simulink model "Aerobic_tank_model"  (R2023a)
settings: Solver=VariableStepAuto  StartTime=0.0  StopTime=10.0  RelTol=1e-3
model workspace (MAT data in the model file):
  Q0 = Simulink.Parameter
  Q0.DataType = 'auto'
  Q0.Complexity = 'real'
  Q0.Dimensions = [0 0]
values from neighbouring files (symbols this model uses):
  iXB = 0.08    [Start2.m]
  iXP = 0.06    [Start2.m]
  kLa = 240    [Start2.m]
  Q1 = 55000    [Start2.m]
  Qa = 10000    [Start2.m]
  Qr = 20000    [Start2.m]
  SALK0 = InputSediments(13)    [Start2.m]
  SALK_ini = 4.93    [Start2.m]
  SALK_ini2 = 4.67    [Start2.m]
  SI0 = InputSediments(1)    [Start2.m]
  SI_ini = 30    [Start2.m]
  SI_ini2 = 30    [Start2.m]
  SND0 = InputSediments(11)    [Start2.m]
  SND_ini = 1.22    [Start2.m]
  SND_ini2 = 0.82    [Start2.m]
  SNH0 = InputSediments(10)    [Start2.m]
  SNH_ini = 7.92    [Start2.m]
  SNH_ini2 = 5.55    [Start2.m]
  SNO0 = InputSediments(9)    [Start2.m]
  SNO_ini = 5.37    [Start2.m]
  SNO_ini2 = 6.54    [Start2.m]
  SO0 = InputSediments(8)    [Start2.m]
  SO_ini = 0.004    [Start2.m]
  SO_ini2 = 1.7    [Start2.m]
  SRT = 100    [Start2.m]
  SS0 = InputSediments(2)    [Start2.m]
  SS_ini = 2.81    [Start2.m]
  SS_ini2 = 1.15    [Start2.m]
  V1 = 1000    [Start2.m]
  XBA0 = InputSediments(6)    [Start2.m]
  XBA_ini = 148    [Start2.m]
  XBA_ini2 = 150    [Start2.m]
  XBH0 = InputSediments(5)    [Start2.m]
  XBH_ini = 2552    [Start2.m]
  XBH_ini2 = 2559    [Start2.m]
  XI0 = InputSediments(3)    [Start2.m]
  XI_ini = 1149    [Start2.m]
  XI_ini2 = 1149    [Start2.m]
  XND0 = InputSediments(12)    [Start2.m]
  XND_ini = 5.28    [Start2.m]
  XND_ini2 = 4.39    [Start2.m]
  XP0 = InputSediments(7)    [Start2.m]
  XP_ini = 449    [Start2.m]
  XP_ini2 = 450    [Start2.m]
  XS0 = InputSediments(4)    [Start2.m]
  XS_ini = 82.1    [Start2.m]
  XS_ini2 = 64.9    [Start2.m]
settings Model: Creator=carlo  LastModifiedBy=carlo

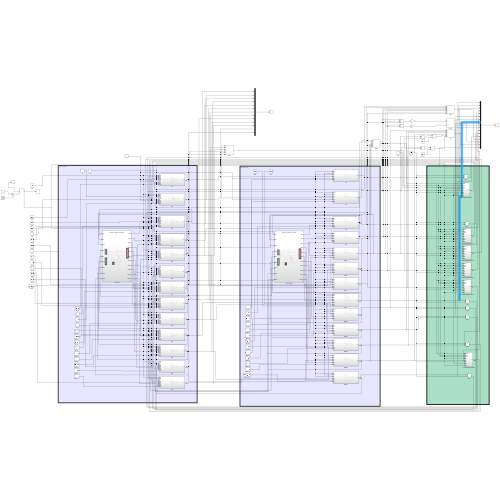
[thumbnail: Simulink's stored preview of the top-level diagram]
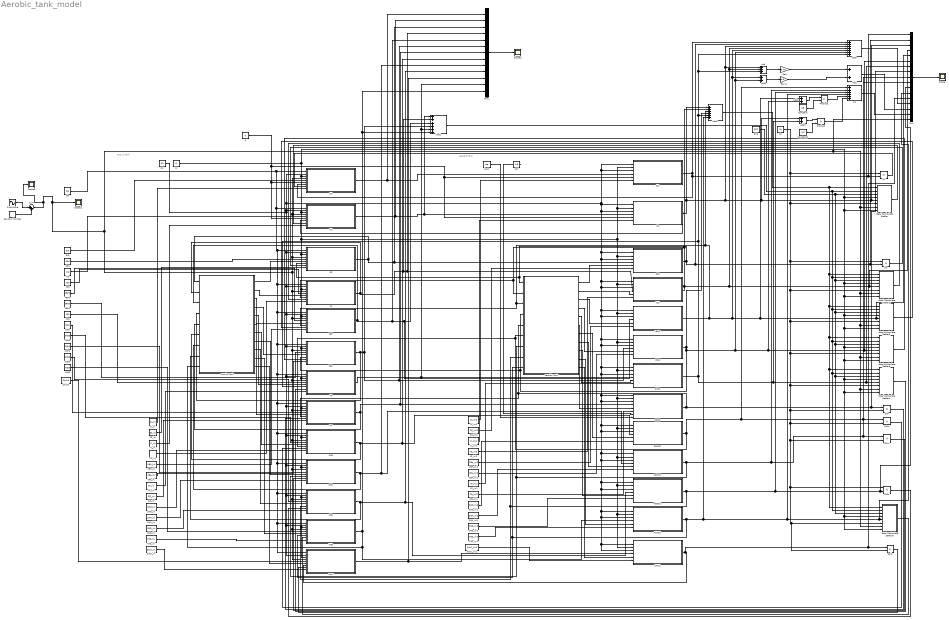
== system Aerobic_tank_model ==
  note: Aerated Tank
  note: Anoxic Tank
  0 : Constant  Value=0
  Add : Sum  Inputs=+++
  Add1 : Sum
  Add2 : Sum
  Add3 : Sum
  Aerobic Tank : Subsystem  ReferencedSubsystem=dynamic_models_processes
  Anoxic Tank : Subsystem  ReferencedSubsystem=dynamic_models_processes
  COD : Sum  Inputs=7
  Constant : Constant  Value=iXB
  Constant1 : Constant  Value=iXP
  Gain : Gain  Gain=0.75
  Gain1 : Gain  Gain=0.9
  Ideal Particulate Settler : Subsystem
  Ideal Particulate Settler1 : Subsystem
  Ideal Particulate Settler2 : Subsystem
  Ideal Particulate Settler3 : Subsystem
  Ideal Particulate Settler4 : Subsystem
  Ideal Particulate Settler5 : Subsystem
  Mux : Mux  Inputs=17
  Mux1 : Mux  Inputs=13
  Product : Product
  Product1 : Product
  Q1 : Constant  Value=Q1
  Qa : Constant  Value=Qa
  Qr : Constant  Value=Qr
  RSND2 : Subsystem
  RSNH2 : Subsystem
  RSNO2 : Subsystem
  RSO2 : Subsystem
  RXND2 : Subsystem
  RXP2 : Subsystem
  Random Number : RandomNumber  Mean=2000  Variance=250000  SampleTime=0.1
  SALK : Subsystem
  SALK0 : Constant  Value=SALK0
  SALK2 : Subsystem
  SALK_ini : Constant  Value=SALK_ini
  SALK_ini1 : Constant  Value=SALK_ini2
  SI0 : Constant  Value=SI0
  SI1 : Subsystem
  SI2 : Subsystem
  SI_ini : Constant  Value=SI_ini
  SI_ini2 : Constant  Value=SI_ini2
  SIr : Product
  SND : Subsystem
  SND0 : Constant  Value=SND0
  SND_ini : Constant  Value=SND_ini
  SND_ini1 : Constant  Value=SND_ini2
  SNDr : Product
  SNH : Subsystem
  SNH0 : Constant  Value=SNH0
  SNH_ini : Constant  Value=SNH_ini
  SNH_ini1 : Constant  Value=SNH_ini2
  SNHr : Product
  SNO : Subsystem
  SNO0 : Constant  Value=SNO0
  SNO_ini : Constant  Value=SNO_ini
  SNO_ini1 : Constant  Value=SNO_ini2
  SNOr : Product
  SO : Subsystem
  SO* : Constant  Value=0.8
  SO0 : Constant  Value=SO0
  SO_ini : Constant  Value=SO_ini
  SO_ini1 : Constant  Value=SO_ini2
  SOr : Product
  SS : Subsystem
  SS0 : Constant  Value=SS0
  SS2 : Subsystem
  SS_ini : Constant  Value=SS_ini
  SS_ini1 : Constant  Value=SS_ini2
  STR : Constant  Value=SRT
  Salkr : Product
  Scope{,1..3} (4 alike) : Scope
  Sine Wave : Sin  Amplitude=10000  Bias=20000  Frequency=2*pi  SampleTime=0
  Ssr : Product
  Sum : Sum  Inputs=|++
  TN : Sum  Inputs=6
  TSS : Sum  Inputs=2
  V1 : Constant  Value=V1
  XBA : Subsystem
  XBA0 : Constant  Value=XBA0
  XBA2 : Subsystem
  XBA_ini : Constant  Value=XBA_ini
  XBA_ini1 : Constant  Value=XBA_ini2
  XBH : Subsystem
  XBH0 : Constant  Value=XBH0
  XBH2 : Subsystem
  XBH_ini : Constant  Value=XBH_ini
  XBH_ini1 : Constant  Value=XBH_ini2
  XI0 : Constant  Value=XI0
  XI1 : Subsystem
  XI2 : Subsystem
  XI_ini : Constant  Value=XI_ini
  XI_ini2 : Constant  Value=XI_ini2
  XND : Subsystem
  XND0 : Constant  Value=XND0
  XND_ini : Constant  Value=XND_ini
  XND_ini1 : Constant  Value=XND_ini2
  XP : Subsystem
  XP0 : Constant  Value=XP0
  XP_ini : Constant  Value=XP_ini
  XP_ini1 : Constant  Value=XP_ini2
  XS : Subsystem
  XS0 : Constant  Value=XS0
  XS2 : Subsystem
  XS_ini : Constant  Value=XS_ini
  XS_ini1 : Constant  Value=XS_ini2
  Xtot1 : Sum  Inputs=6
  Xtot2 : Sum  Inputs=6
  kLa2 : Constant  Value=kLa
  wires:
  V1/1 -> Ideal Particulate Settler1/4(V1), Ideal Particulate Settler3/4(V1), Ideal Particulate Settler3/8(V2), Ideal Particulate Settler5/8(V2), Ideal Particulate Settler5/4(V1), Ideal Particulate Settler4/8(V2), Ideal Particulate Settler4/4(V1), Ideal Particulate Settler2/8(V2), Ideal Particulate Settler2/4(V1), Ideal Particulate Settler1/8(V2), Ideal Particulate Settler/8(V2), Ideal Particulate Settler/4(V1), SNH/3(V1), SALK/3(V1), XND/3(V1), SND/3(V1), SNO/3(V1), SO/3(V1), XP/3(V1), XBA/3(V1), XBH/3(V1), XS/3(V1), SS/3(V1), XI2/2(V2), SI2/2(V2), SALK2/2(V2), RXND2/2(V2), RSND2/2(V2), RSNH2/2(V2), RSNO2/2(V2), RSO2/2(V2), RXP2/2(V2), XBA2/2(V2), XBH2/2(V2), XS2/2(V2), SS2/2(V2), XI1/3(V1), SI1/3(V1)
  Q1/1 -> SALK/2(Q1), XND/2(Q1), SND/2(Q1), SNH/2(Q1), SNO/2(Q1), SO/2(Q1), XP/2(Q1), XBA/2(Q1), XBH/2(Q1), XS/2(Q1), SS/2(Q1), SI1/2(Q1), SS2/3(Q1), SALK2/3(Q1), SALK2/1(Q2), RXND2/3(Q1), RXND2/1(Q2), RSND2/3(Q1), RSND2/1(Q2), RSNH2/3(Q1), RSNH2/1(Q2), RSNO2/3(Q1), RSNO2/1(Q2), RSO2/3(Q1), RSO2/1(Q2), RXP2/3(Q1), RXP2/1(Q2), XBA2/3(Q1), XBA2/1(Q2), XBH2/3(Q1), XBH2/1(Q2), XS2/3(Q1), XS2/1(Q2), SS2/1(Q2), XI2/3(Q1), XI2/1(Q2), SI2/1(Q2), SI2/3(Q1), XI1/2(Q1)
  Sum/1 -> Scope3/1, XBH/4(Q0), SO/4(Q0), SNH/4(Q0), XND/4(Q0), SALK/4(Q0), SND/4(Q0), SNO/4(Q0), XP/4(Q0), XBA/4(Q0), XS/4(Q0), XI1/4(Q0), SI1/4(Q0), SS/4(Q0), Mux/17, Ideal Particulate Settler/7(Q0), Ideal Particulate Settler5/7(Q0), Ideal Particulate Settler4/7(Q0), Ideal Particulate Settler3/7(Q0), Ideal Particulate Settler2/7(Q0), Ideal Particulate Settler1/7(Q0), Scope1/1
  Anoxic Tank/1 -> SS/6(R1)
  SS/1(Z1) -> Mux1/3, SS2/4(Z1), Anoxic Tank/1  "SS1"
  XP0/1 -> XP/5(Z0)
  SNO0/1 -> SNO/5(Z0)
  SND0/1 -> SND/5(Z0)
  SALK0/1 -> SALK/5(Z0)
  Anoxic Tank/2 -> XS/6(R1)
  Anoxic Tank/3 -> XBH/6(R1)
  Anoxic Tank/4 -> XBA/6(R1)
  Anoxic Tank/5 -> XP/6(R1)
  Anoxic Tank/6 -> SO/6(R1)
  Anoxic Tank/7 -> SNO/6(R1)
  Anoxic Tank/8 -> SNH/6(R1)
  Anoxic Tank/9 -> SND/6(R1)
  Anoxic Tank/10 -> XND/6(R1)
  Anoxic Tank/11 -> SALK/6(R1)
  XS/1(Z1) -> Xtot1/2, Mux1/4, XS2/4(Z1), Anoxic Tank/2  "XS1"
  XBH/1(Z1) -> Mux1/5, Xtot1/3, XBH2/4(Z1), Anoxic Tank/3  "XBH1"
  XBA/1(Z1) -> Xtot1/4, Mux1/6, XBA2/4(Z1), Anoxic Tank/4  "XBA1"
  XP/1(Z1) -> RXP2/4(Z1), Mux1/12, Xtot1/5  "XP1"
  SO/1(Z1) -> Anoxic Tank/5, Mux1/7, RSO2/4(Z1)  "SO1"
  SNO/1(Z1) -> Anoxic Tank/6, Mux1/8, RSNO2/4(Z1)  "SNO1"
  SNH/1(Z1) -> Anoxic Tank/7, Mux1/9, RSNH2/4(Z1)  "SNH1"
  SND/1(Z1) -> Anoxic Tank/8, Mux1/10, RSND2/4(Z1)  "SND1"
  XND/1(Z1) -> Mux1/13, Xtot1/6, RXND2/4(Z1), Anoxic Tank/9  "XND1"
  SALK/1(Z1) -> Mux1/11, SALK2/4(Z1)  "SALK1"
  SS_ini/1 -> SS/9(Zini)
  XS_ini/1 -> XS/9(Zini)
  XBH_ini/1 -> XBH/9(Zini)
  XBA_ini/1 -> XBA/9(Zini)
  XP_ini/1 -> XP/9(Zini)
  SO_ini/1 -> SO/9(Zini)
  SNO_ini/1 -> SNO/9(Zini)
  SNH_ini/1 -> SNH/9(Zini)
  SND_ini/1 -> SND/9(Zini)
  XND_ini/1 -> XND/9(Zini)
  SALK_ini/1 -> SALK/9(Zini)
  SS2/1(Z2) -> Mux/2, Ssr/2, COD/2, SS/7(Za), Aerobic Tank/1  "SS2"
  XS2/1(Z2) -> Mux/4, Ideal Particulate Settler1/5(X), Add/2, COD/4, Xtot2/2, XS/7(Za), Aerobic Tank/2
  XBH2/1(Z2) -> Add2/1, Mux/5, Ideal Particulate Settler2/5(X), Add1/1, COD/5, Xtot2/3, XBH/7(Za), Aerobic Tank/3
  XBA2/1(Z2) -> Xtot2/4, XBA/7(Za), Aerobic Tank/4, Add2/2, Ideal Particulate Settler3/5(X), Mux/6, COD/6, Add1/2  "XBA2"
  kLa2/1 -> RSO2/8(kLa)
  SO*/1 -> RSO2/7(SO*)
  RSO2/1(Z2) -> SOr/1, Mux/8, Aerobic Tank/5, SO/7(Za)  "SO2"
  RSNO2/1(Z2) -> TN/1, SNOr/1, Mux/9, Aerobic Tank/6, SNO/7(Za)  "SNO2"
  RSNH2/1(Z2) -> TN/2, SNHr/1, Mux/10, SNH/7(Za), Aerobic Tank/7  "SNH2"
  RSND2/1(Z2) -> TN/3, Mux/11, SNDr/2, SND/7(Za), Aerobic Tank/8  "SND2"
  RXND2/1(Z2) -> Xtot2/6, TN/4, Mux/12, Ideal Particulate Settler5/5(X), XND/7(Za), Aerobic Tank/9  "XND2"
  Aerobic Tank/2 -> XS2/5(R2)
  Aerobic Tank/3 -> XBH2/5(R2)
  Aerobic Tank/4 -> XBA2/5(R2)
  Aerobic Tank/5 -> RXP2/5(R2)
  Aerobic Tank/6 -> RSO2/5(R2)
  Aerobic Tank/7 -> RSNO2/5(R2)
  Aerobic Tank/8 -> RSNH2/5(R2)
  Aerobic Tank/9 -> RSND2/5(R2)
  Aerobic Tank/10 -> RXND2/5(R2)
  Aerobic Tank/11 -> SALK2/5(R2)
  Aerobic Tank/1 -> SS2/5(R2)
  SS_ini1/1 -> SS2/6(Zini)
  XS_ini1/1 -> XS2/6(Zini)
  XBH_ini1/1 -> XBH2/6(Zini)
  XBA_ini1/1 -> XBA2/6(Zini)
  XP_ini1/1 -> RXP2/6(Zini)
  SO_ini1/1 -> RSO2/6(Zini)
  SNO_ini1/1 -> RSNO2/6(Zini)
  SNH_ini1/1 -> RSNH2/6(Zini)
  SND_ini1/1 -> RSND2/6(Zini)
  XND_ini1/1 -> RXND2/6(Zini)
  SALK_ini1/1 -> SALK2/6(Zini)
  SALK2/1(Z2) -> Salkr/1, Mux/13, SALK/7(Za)  "SALK2"
  RXP2/1(Z2) -> Add/3, COD/7, Xtot2/5, XP/7(Za), Add3/2, Ideal Particulate Settler4/5(X), Mux/7  "XP2"
  0/1 -> XI1/6(R1), SI1/6(R1), SI2/5(R2), XI2/5(R2)
  SI0/1 -> SI1/5(Z0)
  SI_ini/1 -> SI1/9(Zini)
  XI_ini/1 -> XI1/9(Zini)
  SI1/1(Z1) -> Mux1/1, SI2/4(Z1)  "SI1"
  XI1/1(Z1) -> Mux1/2, Xtot1/1, XI2/4(Z1)  "XI1"
  SI_ini2/1 -> SI2/6(Zini)
  XI_ini2/1 -> XI2/6(Zini)
  SI2/1(Z2) -> COD/1, SIr/2, Mux/1, SI1/7(Za)
  XI2/1(Z2) -> XI1/7(Za), COD/3, Add/1, Add3/1, Mux/3, Ideal Particulate Settler/5(X), Xtot2/1
  Qr/1 -> Salkr/2, Ideal Particulate Settler5/6(Qr), SNDr/1, SNHr/2, SNOr/2, SOr/2, Ideal Particulate Settler4/6(Qr), Ideal Particulate Settler3/6(Qr), Ideal Particulate Settler2/6(Qr), Ideal Particulate Settler1/6(Qr), Ssr/1, Ideal Particulate Settler/6(Qr), SIr/1
  Xtot2/1 -> Ideal Particulate Settler/1(Xtot2), Ideal Particulate Settler5/1(Xtot2), Ideal Particulate Settler4/1(Xtot2), Ideal Particulate Settler3/1(Xtot2), Ideal Particulate Settler2/1(Xtot2), Ideal Particulate Settler1/1(Xtot2)
  Xtot1/1 -> Ideal Particulate Settler/2(Xtot1), Ideal Particulate Settler5/2(Xtot1), Ideal Particulate Settler4/2(Xtot1), Ideal Particulate Settler3/2(Xtot1), Ideal Particulate Settler2/2(Xtot1), Ideal Particulate Settler1/2(Xtot1)
  STR/1 -> Ideal Particulate Settler/3(STR), Ideal Particulate Settler5/3(STR), Ideal Particulate Settler4/3(STR), Ideal Particulate Settler3/3(STR), Ideal Particulate Settler2/3(STR), Ideal Particulate Settler1/3(STR)
  Ideal Particulate Settler1/1(Zr) -> XS/8(Zr)  "XSr"
  Ideal Particulate Settler2/1(Zr) -> XBH/8(Zr)  "XBHr"
  Ideal Particulate Settler3/1(Zr) -> XBA/8(Zr)  "XBAr"
  Ideal Particulate Settler5/1(Zr) -> XND/8(Zr)  "XNDr"
  SIr/1 -> SI1/8(Zr)
  Ideal Particulate Settler/1(Zr) -> XI1/8(Zr)  "XIr"
  Ssr/1 -> SS/8(Zr)
  Ideal Particulate Settler4/1(Zr) -> XP/8(Zr)  "XPr"
  SOr/1 -> SO/8(Zr)
  SNOr/1 -> SNO/8(Zr)
  SNHr/1 -> SNH/8(Zr)
  SNDr/1 -> SND/8(Zr)
  Salkr/1 -> SALK/8(Zr)
  Qa/1 -> SNH/1(Qa), SALK/1(Qa), XND/1(Qa), SND/1(Qa), SNO/1(Qa), SO/1(Qa), XP/1(Qa), XBA/1(Qa), XBH/1(Qa), XS/1(Qa), SS/1(Qa), XI1/1(Qa), SI1/1(Qa)
  SS0/1 -> SS/5(Z0)
  XI0/1 -> XI1/5(Z0)
  XS0/1 -> XS/5(Z0)
  XBH0/1 -> XBH/5(Z0)
  XBA0/1 -> XBA/5(Z0)
  SO0/1 -> SO/5(Z0)
  SNH0/1 -> SNH/5(Z0)
  XND0/1 -> XND/5(Z0)
  Add/1 -> Gain/1
  Add1/1 -> Gain1/1
  Gain/1 -> TSS/1
  Gain1/1 -> TSS/2
  Constant/1 -> Product1/2
  Add2/1 -> Product1/1
  Product1/1 -> TN/5
  Add3/1 -> Product/1
  Constant1/1 -> Product/2
  Product/1 -> TN/6
  COD/1 -> Mux/14
  TSS/1 -> Mux/15
  TN/1 -> Mux/16
  Mux/1 -> Scope/1
  Mux1/1 -> Scope2/1
  Sine Wave/1 -> Sum/1
  Random Number/1 -> Sum/2

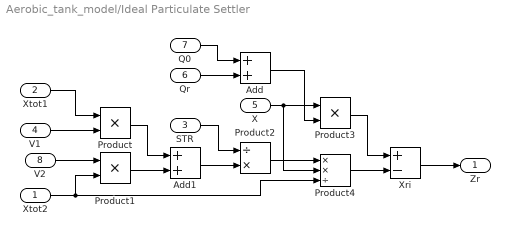
== system Aerobic_tank_model/Ideal Particulate Settler ==
  Xtot2 : Inport
  Xtot1 : Inport  Port=2
  STR : Inport  Port=3
  V1 : Inport  Port=4
  X : Inport  Port=5
  Qr : Inport  Port=6
  Q0 : Inport  Port=7
  V2 : Inport  Port=8
  Add : Sum
  Add1 : Sum
  Product : Product
  Product1 : Product
  Product2 : Product  Inputs=/*
  Product3 : Product
  Product4 : Product  Inputs=**/
  Xri : Sum  Inputs=+-
  Zr : Outport
  wires:
  V1/1 -> Product/2
  Xtot1/1 -> Product/1
  Xtot2/1 -> Product4/3, Product1/2
  STR/1 -> Product2/1
  Q0/1 -> Add/1
  Product/1 -> Add1/1
  Qr/1 -> Add/2
  Product1/1 -> Add1/2
  Add1/1 -> Product2/2
  Add/1 -> Product3/2
  Product4/1 -> Xri/2
  X/1 -> Product3/1, Product4/2
  Product2/1 -> Product4/1
  Product3/1 -> Xri/1
  Xri/1 -> Zr/1
  V2/1 -> Product1/1

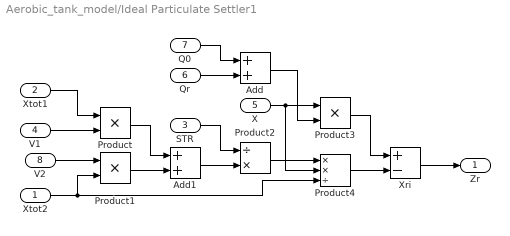
== system Aerobic_tank_model/Ideal Particulate Settler1 ==
  Xtot2 : Inport
  Xtot1 : Inport  Port=2
  STR : Inport  Port=3
  V1 : Inport  Port=4
  X : Inport  Port=5
  Qr : Inport  Port=6
  Q0 : Inport  Port=7
  V2 : Inport  Port=8
  Add : Sum
  Add1 : Sum
  Product : Product
  Product1 : Product
  Product2 : Product  Inputs=/*
  Product3 : Product
  Product4 : Product  Inputs=**/
  Xri : Sum  Inputs=+-
  Zr : Outport
  wires:
  V1/1 -> Product/2
  Xtot1/1 -> Product/1
  Xtot2/1 -> Product4/3, Product1/2
  STR/1 -> Product2/1
  Q0/1 -> Add/1
  Product/1 -> Add1/1
  Qr/1 -> Add/2
  Product1/1 -> Add1/2
  Add1/1 -> Product2/2
  Add/1 -> Product3/2
  Product4/1 -> Xri/2
  X/1 -> Product3/1, Product4/2
  Product2/1 -> Product4/1
  Product3/1 -> Xri/1
  Xri/1 -> Zr/1
  V2/1 -> Product1/1

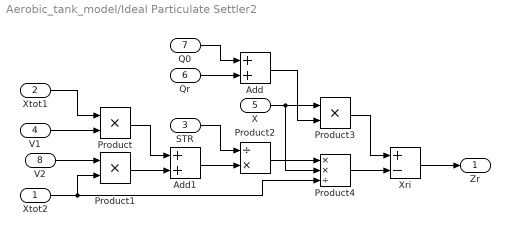
== system Aerobic_tank_model/Ideal Particulate Settler2 ==
  Xtot2 : Inport
  Xtot1 : Inport  Port=2
  STR : Inport  Port=3
  V1 : Inport  Port=4
  X : Inport  Port=5
  Qr : Inport  Port=6
  Q0 : Inport  Port=7
  V2 : Inport  Port=8
  Add : Sum
  Add1 : Sum
  Product : Product
  Product1 : Product
  Product2 : Product  Inputs=/*
  Product3 : Product
  Product4 : Product  Inputs=**/
  Xri : Sum  Inputs=+-
  Zr : Outport
  wires:
  V1/1 -> Product/2
  Xtot1/1 -> Product/1
  Xtot2/1 -> Product4/3, Product1/2
  STR/1 -> Product2/1
  Q0/1 -> Add/1
  Product/1 -> Add1/1
  Qr/1 -> Add/2
  Product1/1 -> Add1/2
  Add1/1 -> Product2/2
  Add/1 -> Product3/2
  Product4/1 -> Xri/2
  X/1 -> Product3/1, Product4/2
  Product2/1 -> Product4/1
  Product3/1 -> Xri/1
  Xri/1 -> Zr/1
  V2/1 -> Product1/1

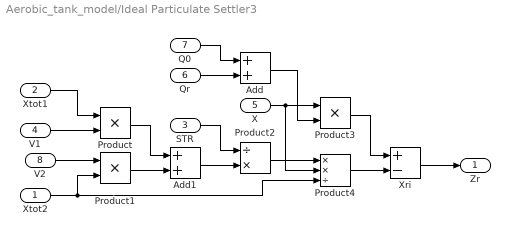
== system Aerobic_tank_model/Ideal Particulate Settler3 ==
  Xtot2 : Inport
  Xtot1 : Inport  Port=2
  STR : Inport  Port=3
  V1 : Inport  Port=4
  X : Inport  Port=5
  Qr : Inport  Port=6
  Q0 : Inport  Port=7
  V2 : Inport  Port=8
  Add : Sum
  Add1 : Sum
  Product : Product
  Product1 : Product
  Product2 : Product  Inputs=/*
  Product3 : Product
  Product4 : Product  Inputs=**/
  Xri : Sum  Inputs=+-
  Zr : Outport
  wires:
  V1/1 -> Product/2
  Xtot1/1 -> Product/1
  Xtot2/1 -> Product4/3, Product1/2
  STR/1 -> Product2/1
  Q0/1 -> Add/1
  Product/1 -> Add1/1
  Qr/1 -> Add/2
  Product1/1 -> Add1/2
  Add1/1 -> Product2/2
  Add/1 -> Product3/2
  Product4/1 -> Xri/2
  X/1 -> Product3/1, Product4/2
  Product2/1 -> Product4/1
  Product3/1 -> Xri/1
  Xri/1 -> Zr/1
  V2/1 -> Product1/1

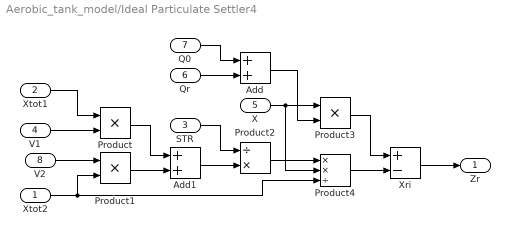
== system Aerobic_tank_model/Ideal Particulate Settler4 ==
  Xtot2 : Inport
  Xtot1 : Inport  Port=2
  STR : Inport  Port=3
  V1 : Inport  Port=4
  X : Inport  Port=5
  Qr : Inport  Port=6
  Q0 : Inport  Port=7
  V2 : Inport  Port=8
  Add : Sum
  Add1 : Sum
  Product : Product
  Product1 : Product
  Product2 : Product  Inputs=/*
  Product3 : Product
  Product4 : Product  Inputs=**/
  Xri : Sum  Inputs=+-
  Zr : Outport
  wires:
  V1/1 -> Product/2
  Xtot1/1 -> Product/1
  Xtot2/1 -> Product4/3, Product1/2
  STR/1 -> Product2/1
  Q0/1 -> Add/1
  Product/1 -> Add1/1
  Qr/1 -> Add/2
  Product1/1 -> Add1/2
  Add1/1 -> Product2/2
  Add/1 -> Product3/2
  Product4/1 -> Xri/2
  X/1 -> Product3/1, Product4/2
  Product2/1 -> Product4/1
  Product3/1 -> Xri/1
  Xri/1 -> Zr/1
  V2/1 -> Product1/1

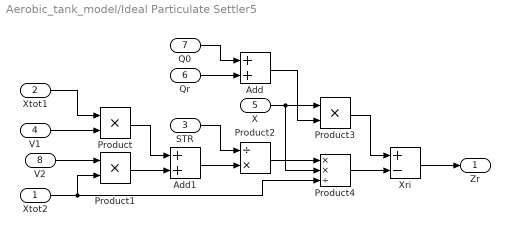
== system Aerobic_tank_model/Ideal Particulate Settler5 ==
  Xtot2 : Inport
  Xtot1 : Inport  Port=2
  STR : Inport  Port=3
  V1 : Inport  Port=4
  X : Inport  Port=5
  Qr : Inport  Port=6
  Q0 : Inport  Port=7
  V2 : Inport  Port=8
  Add : Sum
  Add1 : Sum
  Product : Product
  Product1 : Product
  Product2 : Product  Inputs=/*
  Product3 : Product
  Product4 : Product  Inputs=**/
  Xri : Sum  Inputs=+-
  Zr : Outport
  wires:
  V1/1 -> Product/2
  Xtot1/1 -> Product/1
  Xtot2/1 -> Product4/3, Product1/2
  STR/1 -> Product2/1
  Q0/1 -> Add/1
  Product/1 -> Add1/1
  Qr/1 -> Add/2
  Product1/1 -> Add1/2
  Add1/1 -> Product2/2
  Add/1 -> Product3/2
  Product4/1 -> Xri/2
  X/1 -> Product3/1, Product4/2
  Product2/1 -> Product4/1
  Product3/1 -> Xri/1
  Xri/1 -> Zr/1
  V2/1 -> Product1/1

== system Aerobic_tank_model/RSND2 ==
  Q2 : Inport
  V2 : Inport  Port=2
  Q1 : Inport  Port=3
  Z1 : Inport  Port=4
  R2 : Inport  Port=5
  Zini : Inport  Port=6
  Add : Sum  Inputs=++-
  Integrator : Integrator  InitialConditionSource=external  InitialCondition=SI_ini  ContinuousStateAttributes='SND2'
  Product1 : Product
  Product13 : Product
  Product2 : Product
  Product21 : Product  Inputs=*/
  Z2 : Outport
  wires:
  Product21/1 -> Integrator/1
  Product1/1 -> Add/2
  Integrator/1 -> Z2/1, Product2/1  "SI1"
  Add/1 -> Product21/1
  Product13/1 -> Add/1
  Z1/1 -> Product13/2
  Q2/1 -> Product2/2
  V2/1 -> Product1/1, Product21/2
  Q1/1 -> Product13/1
  R2/1 -> Product1/2
  Zini/1 -> Integrator/2
  Product2/1 -> Add/3

== system Aerobic_tank_model/RSNH2 ==
  Q2 : Inport
  V2 : Inport  Port=2
  Q1 : Inport  Port=3
  Z1 : Inport  Port=4
  R2 : Inport  Port=5
  Zini : Inport  Port=6
  Add : Sum  Inputs=++-
  Integrator : Integrator  InitialConditionSource=external  InitialCondition=SI_ini  ContinuousStateAttributes='SNH2'
  Product1 : Product
  Product13 : Product
  Product2 : Product
  Product21 : Product  Inputs=*/
  Z2 : Outport
  wires:
  Product21/1 -> Integrator/1
  Product1/1 -> Add/2
  Integrator/1 -> Z2/1, Product2/1  "SI1"
  Add/1 -> Product21/1
  Product13/1 -> Add/1
  Z1/1 -> Product13/2
  Q2/1 -> Product2/2
  V2/1 -> Product1/1, Product21/2
  Q1/1 -> Product13/1
  R2/1 -> Product1/2
  Zini/1 -> Integrator/2
  Product2/1 -> Add/3

== system Aerobic_tank_model/RSNO2 ==
  Q2 : Inport
  V2 : Inport  Port=2
  Q1 : Inport  Port=3
  Z1 : Inport  Port=4
  R2 : Inport  Port=5
  Zini : Inport  Port=6
  Add : Sum  Inputs=++-
  Integrator : Integrator  InitialConditionSource=external  InitialCondition=SI_ini  ContinuousStateAttributes='SNO2'
  Product1 : Product
  Product13 : Product
  Product2 : Product
  Product21 : Product  Inputs=*/
  Z2 : Outport
  wires:
  Product21/1 -> Integrator/1
  Product1/1 -> Add/2
  Integrator/1 -> Z2/1, Product2/1  "SI1"
  Add/1 -> Product21/1
  Product13/1 -> Add/1
  Z1/1 -> Product13/2
  Q2/1 -> Product2/2
  V2/1 -> Product1/1, Product21/2
  Q1/1 -> Product13/1
  R2/1 -> Product1/2
  Zini/1 -> Integrator/2
  Product2/1 -> Add/3

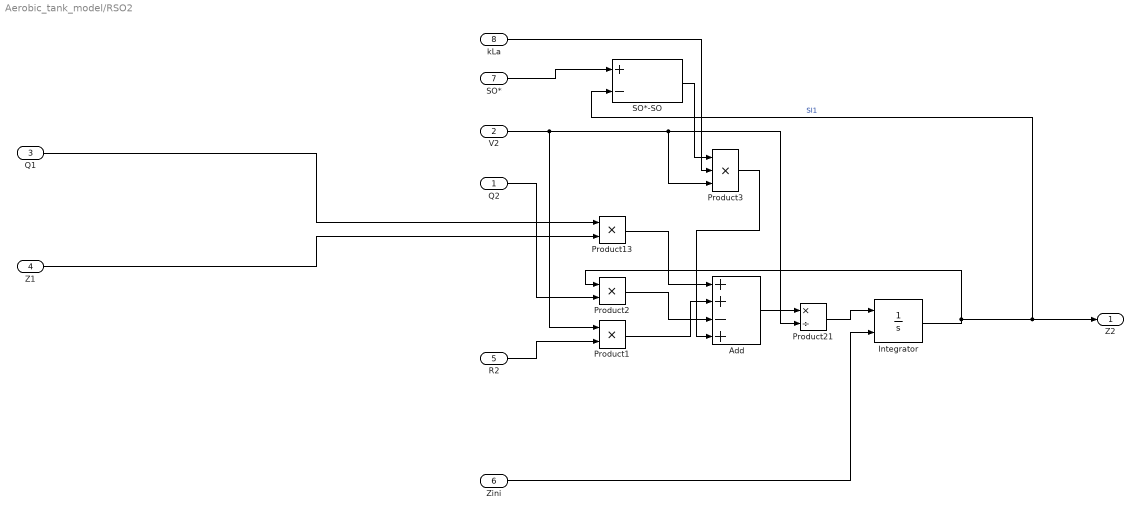
== system Aerobic_tank_model/RSO2 ==
  Q2 : Inport
  V2 : Inport  Port=2
  Q1 : Inport  Port=3
  Z1 : Inport  Port=4
  R2 : Inport  Port=5
  Zini : Inport  Port=6
  SO* : Inport  Port=7
  kLa : Inport  Port=8
  Add : Sum  Inputs=++-+
  Integrator : Integrator  InitialConditionSource=external  InitialCondition=SI_ini  ContinuousStateAttributes='SO2'
  Product1 : Product
  Product13 : Product
  Product2 : Product
  Product21 : Product  Inputs=*/
  Product3 : Product  Inputs=***
  SO*-SO : Sum  Inputs=+-
  Z2 : Outport
  wires:
  Product21/1 -> Integrator/1
  Product1/1 -> Add/2
  Integrator/1 -> SO*-SO/2, Z2/1, Product2/1  "SI1"
  Add/1 -> Product21/1
  Product13/1 -> Add/1
  Z1/1 -> Product13/2
  Q2/1 -> Product2/2
  V2/1 -> Product1/1, Product21/2, Product3/3
  Q1/1 -> Product13/1
  R2/1 -> Product1/2
  Zini/1 -> Integrator/2
  Product2/1 -> Add/3
  SO*/1 -> SO*-SO/1
  SO*-SO/1 -> Product3/1
  kLa/1 -> Product3/2
  Product3/1 -> Add/4

== system Aerobic_tank_model/RXND2 ==
  Q2 : Inport
  V2 : Inport  Port=2
  Q1 : Inport  Port=3
  Z1 : Inport  Port=4
  R2 : Inport  Port=5
  Zini : Inport  Port=6
  Add : Sum  Inputs=++-
  Integrator : Integrator  InitialConditionSource=external  InitialCondition=SI_ini  ContinuousStateAttributes='XND2'
  Product1 : Product
  Product13 : Product
  Product2 : Product
  Product21 : Product  Inputs=*/
  Z2 : Outport
  wires:
  Product21/1 -> Integrator/1
  Product1/1 -> Add/2
  Integrator/1 -> Z2/1, Product2/1  "SI1"
  Add/1 -> Product21/1
  Product13/1 -> Add/1
  Z1/1 -> Product13/2
  Q2/1 -> Product2/2
  V2/1 -> Product1/1, Product21/2
  Q1/1 -> Product13/1
  R2/1 -> Product1/2
  Zini/1 -> Integrator/2
  Product2/1 -> Add/3

== system Aerobic_tank_model/RXP2 ==
  Q2 : Inport
  V2 : Inport  Port=2
  Q1 : Inport  Port=3
  Z1 : Inport  Port=4
  R2 : Inport  Port=5
  Zini : Inport  Port=6
  Add : Sum  Inputs=++-
  Integrator : Integrator  InitialConditionSource=external  InitialCondition=SI_ini  ContinuousStateAttributes='XP2'
  Product1 : Product
  Product13 : Product
  Product2 : Product
  Product21 : Product  Inputs=*/
  Z2 : Outport
  wires:
  Product21/1 -> Integrator/1
  Product1/1 -> Add/2
  Integrator/1 -> Z2/1, Product2/1  "SI1"
  Add/1 -> Product21/1
  Product13/1 -> Add/1
  Z1/1 -> Product13/2
  Q2/1 -> Product2/2
  V2/1 -> Product1/1, Product21/2
  Q1/1 -> Product13/1
  R2/1 -> Product1/2
  Zini/1 -> Integrator/2
  Product2/1 -> Add/3

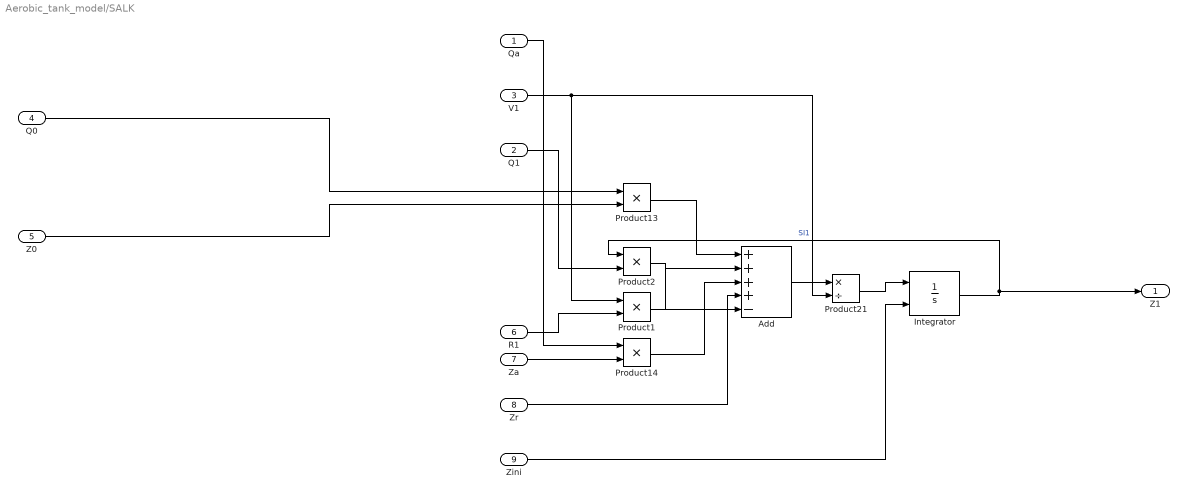
== system Aerobic_tank_model/SALK ==
  Qa : Inport
  Q1 : Inport  Port=2
  V1 : Inport  Port=3
  Q0 : Inport  Port=4
  Z0 : Inport  Port=5
  R1 : Inport  Port=6
  Za : Inport  Port=7
  Zr : Inport  Port=8
  Zini : Inport  Port=9
  Add : Sum  Inputs=++++-
  Integrator : Integrator  InitialConditionSource=external  InitialCondition=SI_ini  ContinuousStateAttributes='SALK1'
  Product{1..2,13..14} (4 alike) : Product
  Product21 : Product  Inputs=*/
  Z1 : Outport
  wires:
  Product21/1 -> Integrator/1
  Product2/1 -> Add/5
  Product1/1 -> Add/2
  Integrator/1 -> Z1/1, Product2/1  "SI1"
  Add/1 -> Product21/1
  Product13/1 -> Add/1
  Qa/1 -> Product14/1
  Z0/1 -> Product13/2
  Zr/1 -> Add/4
  Q1/1 -> Product2/2
  V1/1 -> Product1/1, Product21/2
  Za/1 -> Product14/2
  Q0/1 -> Product13/1
  R1/1 -> Product1/2
  Product14/1 -> Add/3
  Zini/1 -> Integrator/2

== system Aerobic_tank_model/SALK2 ==
  Q2 : Inport
  V2 : Inport  Port=2
  Q1 : Inport  Port=3
  Z1 : Inport  Port=4
  R2 : Inport  Port=5
  Zini : Inport  Port=6
  Add : Sum  Inputs=++-
  Integrator : Integrator  InitialConditionSource=external  InitialCondition=SI_ini  ContinuousStateAttributes='SALK2'
  Product1 : Product
  Product13 : Product
  Product2 : Product
  Product21 : Product  Inputs=*/
  Z2 : Outport
  wires:
  Product21/1 -> Integrator/1
  Product1/1 -> Add/2
  Integrator/1 -> Z2/1, Product2/1  "SI1"
  Add/1 -> Product21/1
  Product13/1 -> Add/1
  Z1/1 -> Product13/2
  Q2/1 -> Product2/2
  V2/1 -> Product1/1, Product21/2
  Q1/1 -> Product13/1
  R2/1 -> Product1/2
  Zini/1 -> Integrator/2
  Product2/1 -> Add/3

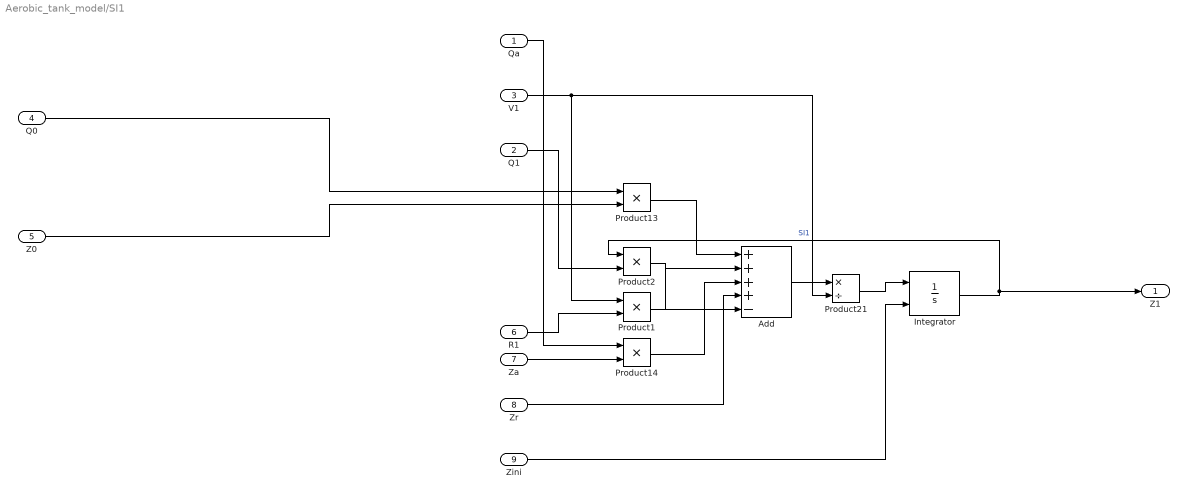
== system Aerobic_tank_model/SI1 ==
  Qa : Inport
  Q1 : Inport  Port=2
  V1 : Inport  Port=3
  Q0 : Inport  Port=4
  Z0 : Inport  Port=5
  R1 : Inport  Port=6
  Za : Inport  Port=7
  Zr : Inport  Port=8
  Zini : Inport  Port=9
  Add : Sum  Inputs=++++-
  Integrator : Integrator  InitialConditionSource=external  InitialCondition=SI_ini  ContinuousStateAttributes='SI1'
  Product{1..2,13..14} (4 alike) : Product
  Product21 : Product  Inputs=*/
  Z1 : Outport
  wires:
  Product21/1 -> Integrator/1
  Product2/1 -> Add/5
  Product1/1 -> Add/2
  Integrator/1 -> Z1/1, Product2/1  "SI1"
  Add/1 -> Product21/1
  Product13/1 -> Add/1
  Qa/1 -> Product14/1
  Z0/1 -> Product13/2
  Q1/1 -> Product2/2
  V1/1 -> Product1/1, Product21/2
  Za/1 -> Product14/2
  Q0/1 -> Product13/1
  R1/1 -> Product1/2
  Product14/1 -> Add/3
  Zr/1 -> Add/4
  Zini/1 -> Integrator/2

== system Aerobic_tank_model/SI2 ==
  Q2 : Inport
  V2 : Inport  Port=2
  Q1 : Inport  Port=3
  Z1 : Inport  Port=4
  R2 : Inport  Port=5
  Zini : Inport  Port=6
  Add : Sum  Inputs=++-
  Integrator : Integrator  InitialConditionSource=external  InitialCondition=SI_ini  ContinuousStateAttributes='SI2'
  Product1 : Product
  Product13 : Product
  Product2 : Product
  Product21 : Product  Inputs=*/
  Z2 : Outport
  wires:
  Product21/1 -> Integrator/1
  Product1/1 -> Add/2
  Integrator/1 -> Z2/1, Product2/1  "SI1"
  Add/1 -> Product21/1
  Product13/1 -> Add/1
  Z1/1 -> Product13/2
  Q2/1 -> Product2/2
  V2/1 -> Product1/1, Product21/2
  Q1/1 -> Product13/1
  R2/1 -> Product1/2
  Zini/1 -> Integrator/2
  Product2/1 -> Add/3

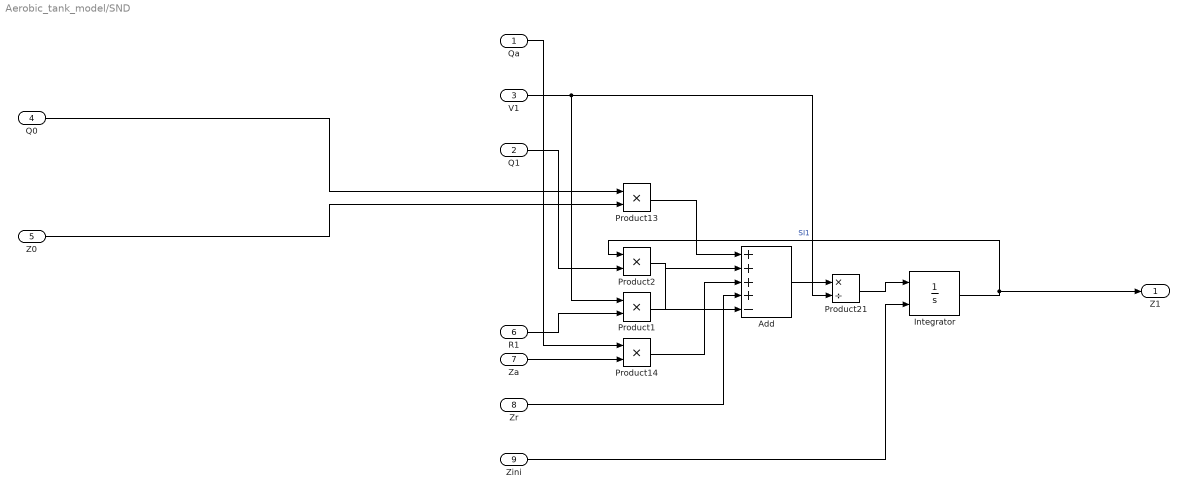
== system Aerobic_tank_model/SND ==
  Qa : Inport
  Q1 : Inport  Port=2
  V1 : Inport  Port=3
  Q0 : Inport  Port=4
  Z0 : Inport  Port=5
  R1 : Inport  Port=6
  Za : Inport  Port=7
  Zr : Inport  Port=8
  Zini : Inport  Port=9
  Add : Sum  Inputs=++++-
  Integrator : Integrator  InitialConditionSource=external  InitialCondition=SI_ini  ContinuousStateAttributes='SND1'
  Product{1..2,13..14} (4 alike) : Product
  Product21 : Product  Inputs=*/
  Z1 : Outport
  wires:
  Product21/1 -> Integrator/1
  Product2/1 -> Add/5
  Product1/1 -> Add/2
  Integrator/1 -> Z1/1, Product2/1  "SI1"
  Add/1 -> Product21/1
  Product13/1 -> Add/1
  Qa/1 -> Product14/1
  Z0/1 -> Product13/2
  Q1/1 -> Product2/2
  V1/1 -> Product1/1, Product21/2
  Za/1 -> Product14/2
  Q0/1 -> Product13/1
  R1/1 -> Product1/2
  Product14/1 -> Add/3
  Zr/1 -> Add/4
  Zini/1 -> Integrator/2

== system Aerobic_tank_model/SNH ==
  Qa : Inport
  Q1 : Inport  Port=2
  V1 : Inport  Port=3
  Q0 : Inport  Port=4
  Z0 : Inport  Port=5
  R1 : Inport  Port=6
  Za : Inport  Port=7
  Zr : Inport  Port=8
  Zini : Inport  Port=9
  Add : Sum  Inputs=++++-
  Integrator : Integrator  InitialConditionSource=external  InitialCondition=SI_ini  ContinuousStateAttributes='SNH1'
  Product{1..2,13..14} (4 alike) : Product
  Product21 : Product  Inputs=*/
  Z1 : Outport
  wires:
  Product21/1 -> Integrator/1
  Product2/1 -> Add/5
  Product1/1 -> Add/2
  Integrator/1 -> Z1/1, Product2/1  "SI1"
  Add/1 -> Product21/1
  Product13/1 -> Add/1
  Qa/1 -> Product14/1
  Z0/1 -> Product13/2
  Q1/1 -> Product2/2
  V1/1 -> Product1/1, Product21/2
  Za/1 -> Product14/2
  Q0/1 -> Product13/1
  R1/1 -> Product1/2
  Product14/1 -> Add/3
  Zr/1 -> Add/4
  Zini/1 -> Integrator/2

== system Aerobic_tank_model/SNO ==
  Qa : Inport
  Q1 : Inport  Port=2
  V1 : Inport  Port=3
  Q0 : Inport  Port=4
  Z0 : Inport  Port=5
  R1 : Inport  Port=6
  Za : Inport  Port=7
  Zr : Inport  Port=8
  Zini : Inport  Port=9
  Add : Sum  Inputs=++++-
  Integrator : Integrator  InitialConditionSource=external  InitialCondition=SI_ini  ContinuousStateAttributes='SNO1'
  Product{1..2,13..14} (4 alike) : Product
  Product21 : Product  Inputs=*/
  Z1 : Outport
  wires:
  Product21/1 -> Integrator/1
  Product2/1 -> Add/5
  Product1/1 -> Add/2
  Integrator/1 -> Z1/1, Product2/1  "SI1"
  Add/1 -> Product21/1
  Product13/1 -> Add/1
  Qa/1 -> Product14/1
  Z0/1 -> Product13/2
  Q1/1 -> Product2/2
  V1/1 -> Product1/1, Product21/2
  Za/1 -> Product14/2
  Q0/1 -> Product13/1
  R1/1 -> Product1/2
  Product14/1 -> Add/3
  Zr/1 -> Add/4
  Zini/1 -> Integrator/2

== system Aerobic_tank_model/SO ==
  Qa : Inport
  Q1 : Inport  Port=2
  V1 : Inport  Port=3
  Q0 : Inport  Port=4
  Z0 : Inport  Port=5
  R1 : Inport  Port=6
  Za : Inport  Port=7
  Zr : Inport  Port=8
  Zini : Inport  Port=9
  Add : Sum  Inputs=++++-
  Integrator : Integrator  InitialConditionSource=external  InitialCondition=SI_ini  ContinuousStateAttributes='SO1'
  Product{1..2,13..14} (4 alike) : Product
  Product21 : Product  Inputs=*/
  Z1 : Outport
  wires:
  Product21/1 -> Integrator/1
  Product2/1 -> Add/5
  Product1/1 -> Add/2
  Integrator/1 -> Z1/1, Product2/1  "SI1"
  Add/1 -> Product21/1
  Product13/1 -> Add/1
  Qa/1 -> Product14/1
  Z0/1 -> Product13/2
  Q1/1 -> Product2/2
  V1/1 -> Product1/1, Product21/2
  Za/1 -> Product14/2
  Q0/1 -> Product13/1
  R1/1 -> Product1/2
  Product14/1 -> Add/3
  Zr/1 -> Add/4
  Zini/1 -> Integrator/2

== system Aerobic_tank_model/SS ==
  Qa : Inport
  Q1 : Inport  Port=2
  V1 : Inport  Port=3
  Q0 : Inport  Port=4
  Z0 : Inport  Port=5
  R1 : Inport  Port=6
  Za : Inport  Port=7
  Zr : Inport  Port=8
  Zini : Inport  Port=9
  Add : Sum  Inputs=++++-
  Integrator : Integrator  InitialConditionSource=external  InitialCondition=SI_ini  ContinuousStateAttributes='SS1'
  Product{1..2,13..14} (4 alike) : Product
  Product21 : Product  Inputs=*/
  Z1 : Outport
  wires:
  Product21/1 -> Integrator/1
  Product2/1 -> Add/5
  Product1/1 -> Add/2
  Integrator/1 -> Z1/1, Product2/1  "SI1"
  Add/1 -> Product21/1
  Product13/1 -> Add/1
  Qa/1 -> Product14/1
  Z0/1 -> Product13/2
  Q1/1 -> Product2/2
  V1/1 -> Product1/1, Product21/2
  Za/1 -> Product14/2
  Q0/1 -> Product13/1
  R1/1 -> Product1/2
  Product14/1 -> Add/3
  Zr/1 -> Add/4
  Zini/1 -> Integrator/2

== system Aerobic_tank_model/SS2 ==
  Q2 : Inport
  V2 : Inport  Port=2
  Q1 : Inport  Port=3
  Z1 : Inport  Port=4
  R2 : Inport  Port=5
  Zini : Inport  Port=6
  Add : Sum  Inputs=++-
  Integrator : Integrator  InitialConditionSource=external  InitialCondition=SI_ini  ContinuousStateAttributes='SS2'
  Product1 : Product
  Product13 : Product
  Product2 : Product
  Product21 : Product  Inputs=*/
  Z2 : Outport
  wires:
  Product21/1 -> Integrator/1
  Product1/1 -> Add/2
  Integrator/1 -> Z2/1, Product2/1  "SI1"
  Add/1 -> Product21/1
  Product13/1 -> Add/1
  Z1/1 -> Product13/2
  Q2/1 -> Product2/2
  V2/1 -> Product1/1, Product21/2
  Q1/1 -> Product13/1
  R2/1 -> Product1/2
  Zini/1 -> Integrator/2
  Product2/1 -> Add/3

== system Aerobic_tank_model/XBA ==
  Qa : Inport
  Q1 : Inport  Port=2
  V1 : Inport  Port=3
  Q0 : Inport  Port=4
  Z0 : Inport  Port=5
  R1 : Inport  Port=6
  Za : Inport  Port=7
  Zr : Inport  Port=8
  Zini : Inport  Port=9
  Add : Sum  Inputs=++++-
  Integrator : Integrator  InitialConditionSource=external  InitialCondition=SI_ini  ContinuousStateAttributes='XBA1'
  Product{1..2,13..14} (4 alike) : Product
  Product21 : Product  Inputs=*/
  Z1 : Outport
  wires:
  Product21/1 -> Integrator/1
  Product2/1 -> Add/5
  Product1/1 -> Add/2
  Integrator/1 -> Z1/1, Product2/1  "SI1"
  Add/1 -> Product21/1
  Product13/1 -> Add/1
  Qa/1 -> Product14/1
  Z0/1 -> Product13/2
  Q1/1 -> Product2/2
  V1/1 -> Product1/1, Product21/2
  Za/1 -> Product14/2
  Q0/1 -> Product13/1
  R1/1 -> Product1/2
  Product14/1 -> Add/3
  Zr/1 -> Add/4
  Zini/1 -> Integrator/2

== system Aerobic_tank_model/XBA2 ==
  Q2 : Inport
  V2 : Inport  Port=2
  Q1 : Inport  Port=3
  Z1 : Inport  Port=4
  R2 : Inport  Port=5
  Zini : Inport  Port=6
  Add : Sum  Inputs=++-
  Integrator : Integrator  InitialConditionSource=external  InitialCondition=SI_ini  ContinuousStateAttributes='XBA2'
  Product1 : Product
  Product13 : Product
  Product2 : Product
  Product21 : Product  Inputs=*/
  Z2 : Outport
  wires:
  Product21/1 -> Integrator/1
  Product1/1 -> Add/2
  Integrator/1 -> Z2/1, Product2/1  "SI1"
  Add/1 -> Product21/1
  Product13/1 -> Add/1
  Z1/1 -> Product13/2
  Q2/1 -> Product2/2
  V2/1 -> Product1/1, Product21/2
  Q1/1 -> Product13/1
  R2/1 -> Product1/2
  Zini/1 -> Integrator/2
  Product2/1 -> Add/3

== system Aerobic_tank_model/XBH ==
  Qa : Inport
  Q1 : Inport  Port=2
  V1 : Inport  Port=3
  Q0 : Inport  Port=4
  Z0 : Inport  Port=5
  R1 : Inport  Port=6
  Za : Inport  Port=7
  Zr : Inport  Port=8
  Zini : Inport  Port=9
  Add : Sum  Inputs=++++-
  Integrator : Integrator  InitialConditionSource=external  InitialCondition=SI_ini  ContinuousStateAttributes='XBH1'
  Product{1..2,13..14} (4 alike) : Product
  Product21 : Product  Inputs=*/
  Z1 : Outport
  wires:
  Product21/1 -> Integrator/1
  Product2/1 -> Add/5
  Product1/1 -> Add/2
  Integrator/1 -> Z1/1, Product2/1  "SI1"
  Add/1 -> Product21/1
  Product13/1 -> Add/1
  Qa/1 -> Product14/1
  Z0/1 -> Product13/2
  Q1/1 -> Product2/2
  V1/1 -> Product1/1, Product21/2
  Za/1 -> Product14/2
  Q0/1 -> Product13/1
  R1/1 -> Product1/2
  Product14/1 -> Add/3
  Zr/1 -> Add/4
  Zini/1 -> Integrator/2

== system Aerobic_tank_model/XBH2 ==
  Q2 : Inport
  V2 : Inport  Port=2
  Q1 : Inport  Port=3
  Z1 : Inport  Port=4
  R2 : Inport  Port=5
  Zini : Inport  Port=6
  Add : Sum  Inputs=++-
  Integrator : Integrator  InitialConditionSource=external  InitialCondition=SI_ini  ContinuousStateAttributes='XBH2'
  Product1 : Product
  Product13 : Product
  Product2 : Product
  Product21 : Product  Inputs=*/
  Z2 : Outport
  wires:
  Product21/1 -> Integrator/1
  Product1/1 -> Add/2
  Integrator/1 -> Z2/1, Product2/1  "SI1"
  Add/1 -> Product21/1
  Product13/1 -> Add/1
  Z1/1 -> Product13/2
  Q2/1 -> Product2/2
  V2/1 -> Product1/1, Product21/2
  Q1/1 -> Product13/1
  R2/1 -> Product1/2
  Zini/1 -> Integrator/2
  Product2/1 -> Add/3

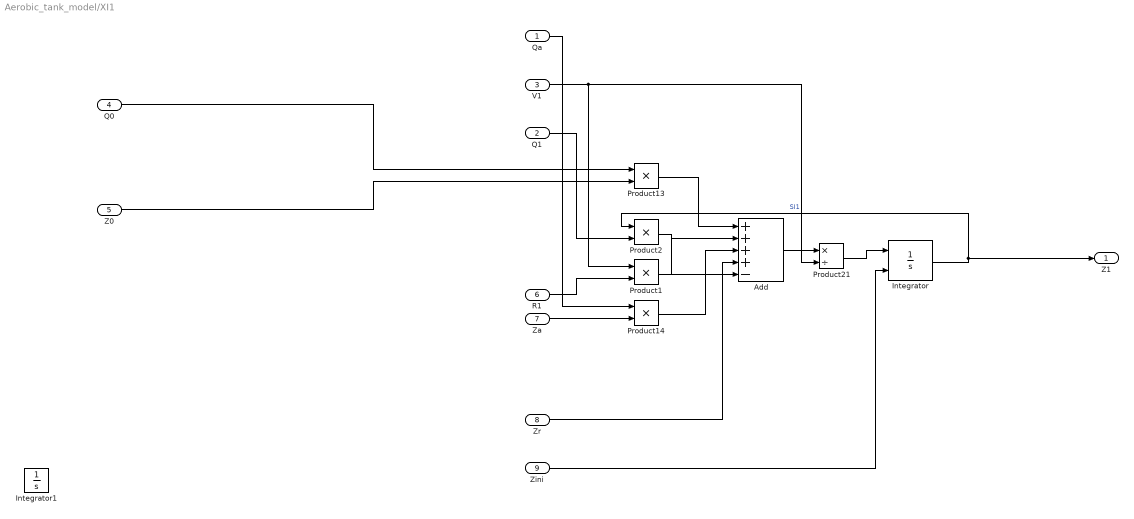
== system Aerobic_tank_model/XI1 ==
  Qa : Inport
  Q1 : Inport  Port=2
  V1 : Inport  Port=3
  Q0 : Inport  Port=4
  Z0 : Inport  Port=5
  R1 : Inport  Port=6
  Za : Inport  Port=7
  Zr : Inport  Port=8
  Zini : Inport  Port=9
  Add : Sum  Inputs=++++-
  Integrator : Integrator  InitialConditionSource=external  InitialCondition=SI_ini  ContinuousStateAttributes='XI1'
  Integrator1 : Integrator
  Product{1..2,13..14} (4 alike) : Product
  Product21 : Product  Inputs=*/
  Z1 : Outport
  wires:
  Product21/1 -> Integrator/1
  Product2/1 -> Add/5
  Product1/1 -> Add/2
  Integrator/1 -> Z1/1, Product2/1  "SI1"
  Add/1 -> Product21/1
  Product13/1 -> Add/1
  Qa/1 -> Product14/1
  Z0/1 -> Product13/2
  Q1/1 -> Product2/2
  V1/1 -> Product1/1, Product21/2
  Za/1 -> Product14/2
  Q0/1 -> Product13/1
  R1/1 -> Product1/2
  Product14/1 -> Add/3
  Zr/1 -> Add/4
  Zini/1 -> Integrator/2

== system Aerobic_tank_model/XI2 ==
  Q2 : Inport
  V2 : Inport  Port=2
  Q1 : Inport  Port=3
  Z1 : Inport  Port=4
  R2 : Inport  Port=5
  Zini : Inport  Port=6
  Add : Sum  Inputs=++-
  Integrator : Integrator  InitialConditionSource=external  InitialCondition=SI_ini  ContinuousStateAttributes='XI2'
  Product1 : Product
  Product13 : Product
  Product2 : Product
  Product21 : Product  Inputs=*/
  Z2 : Outport
  wires:
  Product21/1 -> Integrator/1
  Product1/1 -> Add/2
  Integrator/1 -> Z2/1, Product2/1  "SI1"
  Add/1 -> Product21/1
  Product13/1 -> Add/1
  Z1/1 -> Product13/2
  Q2/1 -> Product2/2
  V2/1 -> Product1/1, Product21/2
  Q1/1 -> Product13/1
  R2/1 -> Product1/2
  Zini/1 -> Integrator/2
  Product2/1 -> Add/3

== system Aerobic_tank_model/XND ==
  Qa : Inport
  Q1 : Inport  Port=2
  V1 : Inport  Port=3
  Q0 : Inport  Port=4
  Z0 : Inport  Port=5
  R1 : Inport  Port=6
  Za : Inport  Port=7
  Zr : Inport  Port=8
  Zini : Inport  Port=9
  Add : Sum  Inputs=++++-
  Integrator : Integrator  InitialConditionSource=external  InitialCondition=SI_ini  ContinuousStateAttributes='XND1'
  Product{1..2,13..14} (4 alike) : Product
  Product21 : Product  Inputs=*/
  Z1 : Outport
  wires:
  Product21/1 -> Integrator/1
  Product2/1 -> Add/5
  Product1/1 -> Add/2
  Integrator/1 -> Z1/1, Product2/1  "SI1"
  Add/1 -> Product21/1
  Product13/1 -> Add/1
  Qa/1 -> Product14/1
  Z0/1 -> Product13/2
  Q1/1 -> Product2/2
  V1/1 -> Product1/1, Product21/2
  Za/1 -> Product14/2
  Q0/1 -> Product13/1
  R1/1 -> Product1/2
  Product14/1 -> Add/3
  Zr/1 -> Add/4
  Zini/1 -> Integrator/2

== system Aerobic_tank_model/XP ==
  Qa : Inport
  Q1 : Inport  Port=2
  V1 : Inport  Port=3
  Q0 : Inport  Port=4
  Z0 : Inport  Port=5
  R1 : Inport  Port=6
  Za : Inport  Port=7
  Zr : Inport  Port=8
  Zini : Inport  Port=9
  Add : Sum  Inputs=++++-
  Integrator : Integrator  InitialConditionSource=external  InitialCondition=SI_ini  ContinuousStateAttributes='XP1'
  Product{1..2,13..14} (4 alike) : Product
  Product21 : Product  Inputs=*/
  Z1 : Outport
  wires:
  Product21/1 -> Integrator/1
  Product2/1 -> Add/5
  Product1/1 -> Add/2
  Integrator/1 -> Z1/1, Product2/1  "SI1"
  Add/1 -> Product21/1
  Product13/1 -> Add/1
  Qa/1 -> Product14/1
  Z0/1 -> Product13/2
  Q1/1 -> Product2/2
  V1/1 -> Product1/1, Product21/2
  Za/1 -> Product14/2
  Q0/1 -> Product13/1
  R1/1 -> Product1/2
  Product14/1 -> Add/3
  Zr/1 -> Add/4
  Zini/1 -> Integrator/2

== system Aerobic_tank_model/XS ==
  Qa : Inport
  Q1 : Inport  Port=2
  V1 : Inport  Port=3
  Q0 : Inport  Port=4
  Z0 : Inport  Port=5
  R1 : Inport  Port=6
  Za : Inport  Port=7
  Zr : Inport  Port=8
  Zini : Inport  Port=9
  Add : Sum  Inputs=++++-
  Integrator : Integrator  InitialConditionSource=external  InitialCondition=SI_ini  ContinuousStateAttributes='XS1'
  Product{1..2,13..14} (4 alike) : Product
  Product21 : Product  Inputs=*/
  Z1 : Outport
  wires:
  Product21/1 -> Integrator/1
  Product2/1 -> Add/5
  Product1/1 -> Add/2
  Integrator/1 -> Z1/1, Product2/1  "SI1"
  Add/1 -> Product21/1
  Product13/1 -> Add/1
  Qa/1 -> Product14/1
  Z0/1 -> Product13/2
  Q1/1 -> Product2/2
  V1/1 -> Product1/1, Product21/2
  Za/1 -> Product14/2
  Q0/1 -> Product13/1
  R1/1 -> Product1/2
  Product14/1 -> Add/3
  Zr/1 -> Add/4
  Zini/1 -> Integrator/2

== system Aerobic_tank_model/XS2 ==
  Q2 : Inport
  V2 : Inport  Port=2
  Q1 : Inport  Port=3
  Z1 : Inport  Port=4
  R2 : Inport  Port=5
  Zini : Inport  Port=6
  Add : Sum  Inputs=++-
  Integrator : Integrator  InitialConditionSource=external  InitialCondition=SI_ini  ContinuousStateAttributes='XS2'
  Product1 : Product
  Product13 : Product
  Product2 : Product
  Product21 : Product  Inputs=*/
  Z2 : Outport
  wires:
  Product21/1 -> Integrator/1
  Product1/1 -> Add/2
  Integrator/1 -> Z2/1, Product2/1  "SI1"
  Add/1 -> Product21/1
  Product13/1 -> Add/1
  Z1/1 -> Product13/2
  Q2/1 -> Product2/2
  V2/1 -> Product1/1, Product21/2
  Q1/1 -> Product13/1
  R2/1 -> Product1/2
  Zini/1 -> Integrator/2
  Product2/1 -> Add/3
